simulink model "pidgantrycraneV"  (R2021a)
settings: Solver=VariableStepAuto  StartTime=0.0  StopTime=10  RelTol=1e-3
libraries: vrlib x3
settings Model: Creator=khoi  LastModifiedBy=khoi

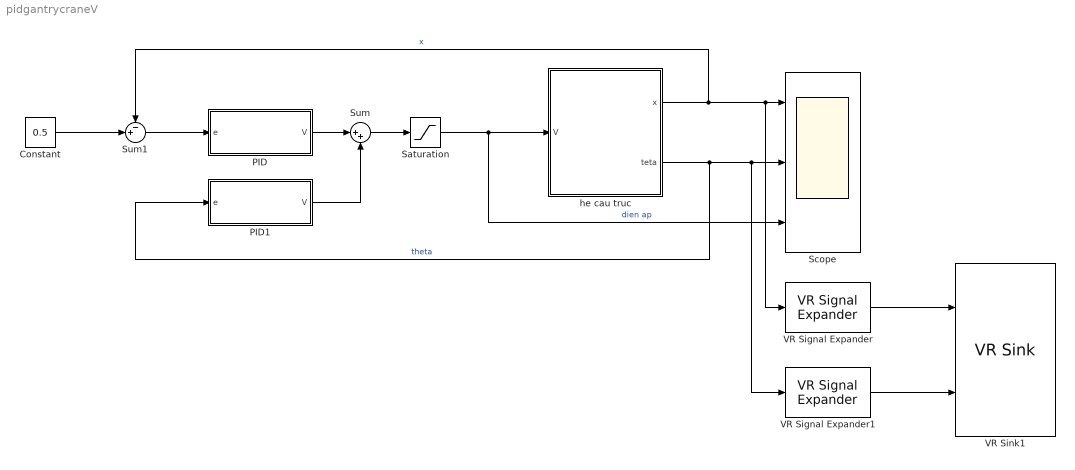
== system pidgantrycraneV ==
  Constant : Constant  Value=0.5
  PID : Subsystem
  PID1 : Subsystem
  Saturation : Saturate  UpperLimit=12  LowerLimit=-12
  Scope : Scope  NumInputPorts=3
  Sum : Sum  Inputs=|++
  Sum1 : Sum  Inputs=-+|
  VR Signal Expander : vrlib/VR Signal Expander  outwidth=3  outidx=[1]
  VR Signal Expander1 : vrlib/VR Signal Expander  outwidth=4  outidx=[4]
  VR Sink1 : vrlib/VR Sink  InstantiateOnLoad=on  SampleTime=0.1  ViewEnable=on  RemoteChange=off  RemoteView=off  FieldsWritten=xe.translation.3.1.1.double#goc.rotation.4.1.1.double  WorldFileName=crane.x3d  AutoView=off  VideoDimensions=[]  AllowVariableSize=off
  he cau truc : Subsystem
  wires:
  VR Signal Expander/1 -> VR Sink1/1
  PID/1(V) -> Sum/1
  Constant/1 -> Sum1/2
  he cau truc/2(teta) -> VR Signal Expander1/1, Scope/2, PID1/1(e)  "theta"
  PID1/1(V) -> Sum/2
  he cau truc/1(x) -> VR Signal Expander/1, Scope/1, Sum1/1  "x"
  VR Signal Expander1/1 -> VR Sink1/2
  Saturation/1 -> Scope/3, he cau truc/1(V)  "dien ap"
  Sum/1 -> Saturation/1
  Sum1/1 -> PID/1(e)

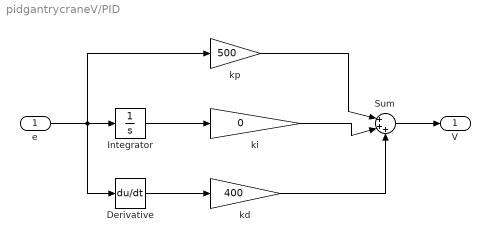
== system pidgantrycraneV/PID ==
  e : Inport
  Derivative : Derivative
  Integrator : Integrator
  Sum : Sum  Inputs=|+++
  kd : Gain  Gain=400
  ki : Gain  Gain=0
  kp : Gain  Gain=500
  V : Outport
  wires:
  Integrator/1 -> ki/1
  Derivative/1 -> kd/1
  ki/1 -> Sum/2
  kp/1 -> Sum/1
  kd/1 -> Sum/3
  Sum/1 -> V/1
  e/1 -> Derivative/1, kp/1, Integrator/1

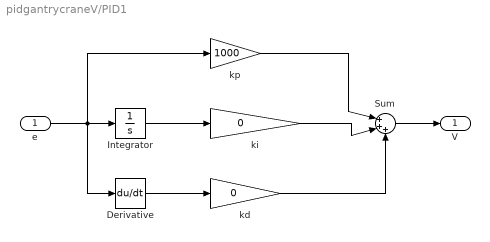
== system pidgantrycraneV/PID1 ==
  e : Inport
  Derivative : Derivative
  Integrator : Integrator
  Sum : Sum  Inputs=|+++
  kd : Gain  Gain=0
  ki : Gain  Gain=0
  kp : Gain  Gain=1000
  V : Outport
  wires:
  Integrator/1 -> ki/1
  Derivative/1 -> kd/1
  ki/1 -> Sum/2
  kp/1 -> Sum/1
  kd/1 -> Sum/3
  Sum/1 -> V/1
  e/1 -> Derivative/1, kp/1, Integrator/1

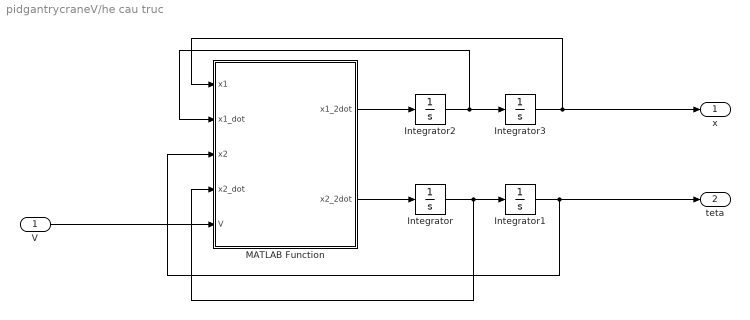
== system pidgantrycraneV/he cau truc ==
  V : Inport
  Integrator{,1..3} (4 alike) : Integrator
  MATLAB Function : MATLAB Function  TreatAsAtomicUnit=on
  x : Outport
  teta : Outport  Port=2
  wires:
  V/1 -> MATLAB Function/5(V)
  MATLAB Function/2(x2_2dot) -> Integrator/1
  Integrator3/1 -> x/1, MATLAB Function/1(x1)
  Integrator/1 -> MATLAB Function/4(x2_dot), Integrator1/1
  Integrator2/1 -> Integrator3/1, MATLAB Function/2(x1_dot)
  MATLAB Function/1(x1_2dot) -> Integrator2/1
  Integrator1/1 -> teta/1, MATLAB Function/3(x2)

== matlab function pidgantrycraneV/he cau truc/MATLAB Function ==
  data: x1 input; x1_dot input; x1_2dot output; x2_2dot output; x2 input; x2_dot input; V input
function [x1_2dot,x2_2dot] = fcn(x1,x1_dot,x2,x2_dot,V)
m1=1;m2=5;l=0.75;g=9.81;B=123.2;R=2.6;KT=0.007;KE=0.007;rp=0.02;z=15;

x1_2dot =(KT*V*rp*z - KE*KT*x1_dot*z^2 - B*R*rp^2*x1_dot + R*g*m1*rp^2*cos(x2)*sin(x2) + R*l*m1*rp^2*x2_dot^2*sin(x2))/(R*rp^2*(- m1*cos(x2)^2 + m1 + m2));
 
 
x2_2dot =-(R*g*m1*rp^2*sin(x2) - KE*KT*x1_dot*z^2*cos(x2) - B*R*rp^2*x1_dot*cos(x2) + R*g*m2*rp^2*sin(x2) + KT*V*rp*z*cos(x2) + R*l*m1*rp^2*x2_dot^2*cos(x2)*sin(x2))/(R*l*rp^2*(- m1*cos(x2)^2 + m1 + m2));
